simulink model "pid_nco_org"  (R2018a)
settings: Solver=VariableStepAuto  StartTime=0.0  StopTime=10000  RelTol=1e-3
undefined symbols (not defined in the file): coeff, RadioSampleRate
libraries: RxTxFixedPointLibrary_noscopes_mod x2, commsource2 x1, dsphdlfiltering x1
settings Model: Creator=czjte  LastModifiedBy=czjte

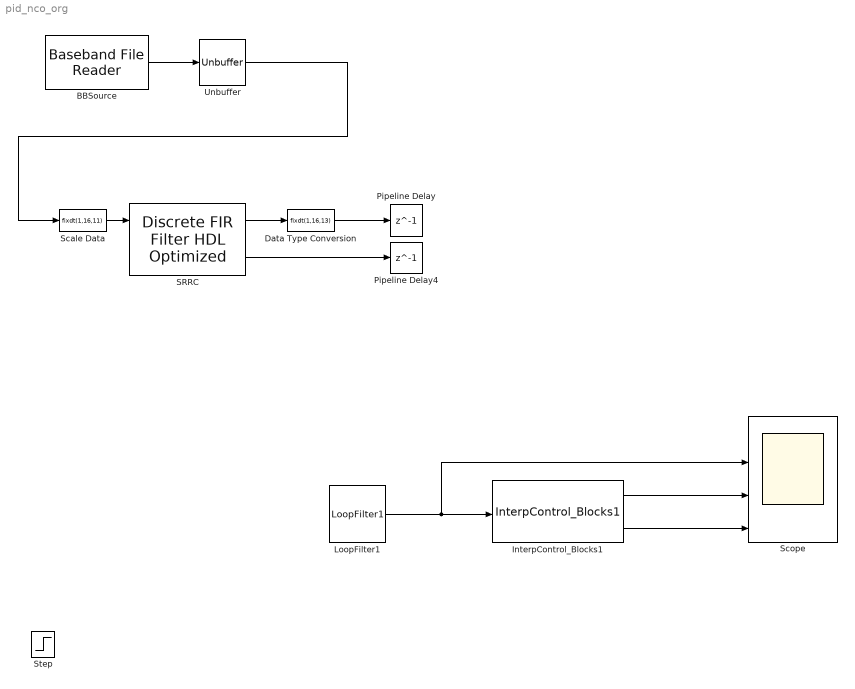
== system pid_nco_org ==
  BBSource : commsource2/Baseband File Reader  Filename=PlutoCaptureQPSK.bb  InheritSampleTimeFromFile=off  SampleTime=100000/(RadioSampleRate)  SamplesPerFrame=100000  CyclicRepetition=off  FileEndOutputPort=off  SimulateUsing=Interpreted execution
      settings: SourceProductName=Communications System Toolbox  SourceProductBaseCode=CM
  Data Type Conversion : DataTypeConversion  OutDataTypeStr=fixdt(1,16,13)
  InterpControl_Blocks1 : RxTxFixedPointLibrary_noscopes_mod/Receiver HDL/Frame Recover/Gardner Timing Recovery/InterpControl_Blocks1
  LoopFilter1 : RxTxFixedPointLibrary_noscopes_mod/Receiver HDL/Frame Recover/Gardner Timing Recovery/LoopFilter1  zeta=sqrt(2)  BnTs=0.01  Kp=2.7
  Pipeline Delay : Delay  DelayLength=1
  Pipeline Delay4 : Delay  DelayLength=1
  SRRC : dsphdlfiltering/Discrete FIR Filter HDL Optimized  Numerator=coeff  Sharing=off  SharingFactor=2  SimulateUsing=Code generation  roundingMode=Floor  overflowMode=on  CoefficientsDataTypeStr=Inherit: Same word length as input  CoefficientsMin=[]  CoefficientsMax=[]  OutputDataTypeStr=fixdt(1,16,11)  OutputMin=[]  OutputMax=[]  ValidInPort=on  ReadyPort=off
      settings: SourceProductName=DSP System Toolbox  SourceProductBaseCode=DS
  Scale Data : DataTypeConversion  OutDataTypeStr=fixdt(1,16,11)  ConvertRealWorld=Stored Integer (SI)  SaturateOnIntegerOverflow=on
  Scope : Scope  NumInputPorts=4
  Step : Step  Time=0.01  After=2  SampleTime=0
  Unbuffer : Unbuffer
  wires:
  LoopFilter1/1 -> Scope/2, InterpControl_Blocks1/1
  ? -> Scope/1, LoopFilter1/1
  InterpControl_Blocks1/1 -> Scope/3
  InterpControl_Blocks1/2 -> Scope/4
  BBSource/1 -> Unbuffer/1
  SRRC/1 -> Data Type Conversion/1
  Scale Data/1 -> SRRC/1
  Unbuffer/1 -> Scale Data/1
  Data Type Conversion/1 -> Pipeline Delay/1
  SRRC/2 -> Pipeline Delay4/1
